simulink model "hvac2"  (R2014a)
settings: Solver=ode45  StartTime=0.0  StopTime=inf  RelTol=1e-3
settings Model: Creator=feisele  LastModifiedBy=feisele

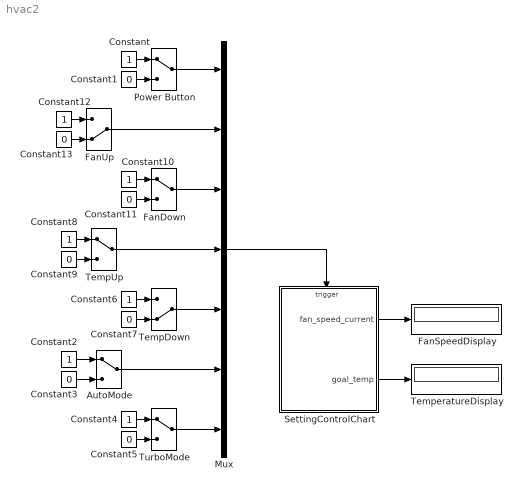
== system hvac2 ==
  AutoMode : ManualSwitch
  Constant{,2,4,6,8,10,12} (7 alike) : Constant
  Constant{1,3,5,7,9,11,13} (7 alike) : Constant  Value=0
  FanDown : ManualSwitch
  FanSpeedDisplay : Display
  FanUp : ManualSwitch  CurrentSetting=0
  Mux : Mux  Inputs=7
  Power Button : ManualSwitch
  SettingControlChart : Stateflow chart  TreatAsAtomicUnit=on
  TempDown : ManualSwitch  CurrentSetting=0
  TempUp : ManualSwitch
  TemperatureDisplay : Display
  TurboMode : ManualSwitch
  wires:
  Power Button/1 -> Mux/1
  Constant/1 -> Power Button/1
  SettingControlChart/1(fan_speed_current) -> FanSpeedDisplay/1
  SettingControlChart/2(goal_temp) -> TemperatureDisplay/1
  FanUp/1 -> Mux/2
  Mux/1 -> SettingControlChart/Trigger
  FanDown/1 -> Mux/3
  TempUp/1 -> Mux/4
  TempDown/1 -> Mux/5
  Constant2/1 -> AutoMode/1
  Constant3/1 -> AutoMode/2
  Constant4/1 -> TurboMode/1
  Constant5/1 -> TurboMode/2
  AutoMode/1 -> Mux/6
  TurboMode/1 -> Mux/7
  Constant6/1 -> TempDown/1
  Constant7/1 -> TempDown/2
  Constant8/1 -> TempUp/1
  Constant9/1 -> TempUp/2
  Constant10/1 -> FanDown/1
  Constant11/1 -> FanDown/2
  Constant12/1 -> FanUp/1
  Constant13/1 -> FanUp/2
  Constant1/1 -> Power Button/2

== stateflow chart hvac2/SettingControlChart ==
  settings: executeAtInitialization=1
  state Power_on
    state Fan_setting [parallel]
      settings: executionOrder=2
      state Fan
      Fan -> Fan [order 1] : fan_up [fan_speed_current < MAXF]
          | { manual_fan = manual_fan + 1;
          | manual_on }
      (default) -> Fan
      Fan -> Fan [order 2] : fan_down [MINF < fan_speed_current]
          | { manual_fan = manual_fan - 1;
          | manual_on }
    state Temperature_setting [parallel]
      settings: executionOrder=1
      state Temp
      Temp -> Temp [order 1] : temp_up [goal_temp < MAXT]
          | { manual_temp = manual_temp + 1;
          | goal_temp = manual_temp; }
      (default) -> Temp : { goal_temp = manual_temp; }
      Temp -> Temp [order 2] : temp_down [MINT < goal_temp]
          | { manual_temp = manual_temp - 1;
          | goal_temp = manual_temp; }
    state Mode_setting [parallel]
      settings: executionOrder=3
      (history)
      state ManualMode
      state Computed_mode
        (history)
        state Auto_mode
        state Turboo_mode
        (default) -> Auto_mode : { fan_speed_current = AUTO_FAN; }
      ManualMode -> ManualMode : manual_on
          | { fan_speed_current = manual_fan; }
      Computed_mode -> ManualMode : manual_on
          | { fan_speed_current = manual_fan;
          | goal_temp = manual_temp; }
      (default) -> Computed_mode
      Mode_setting -> Auto_mode [order 2] : auto_on
          | { fan_speed_current = AUTO_FAN;
          | goal_temp = manual_temp; }
      Mode_setting -> Turboo_mode [order 1] : turbo_on
          | { fan_speed_current = MAXF;
          | goal_temp = MAXT; }
  state Power_off
  Power_off -> Power_on : power_press
  (default) -> Power_off : {manual_fan = int8(5);
      |  manual_temp = int8(10); }
  Power_on -> Power_off : power_press
  data: MAXF constant int8 =10; MINF constant int8 =0; MINT constant int8 =0; MAXT constant int8 =30; fan_speed_current output int8; goal_temp output int8; manual_fan local int8 =5; manual_temp local int8 =10; AUTO_FAN constant int8 =7
  events: power_press input EITHER_EDGE_EVENT; manual_on local FUNCTION_CALL_EVENT; fan_up input EITHER_EDGE_EVENT; fan_down input EITHER_EDGE_EVENT; temp_up input EITHER_EDGE_EVENT; temp_down input EITHER_EDGE_EVENT; auto_on input EITHER_EDGE_EVENT; turbo_on input EITHER_EDGE_EVENT
